simulink model "bus"  (R2020a)
settings: Solver=ode45  StartTime=0.0  StopTime=10.0  RelTol=1e-3
settings Model: Creator=11973  LastModifiedBy=11973

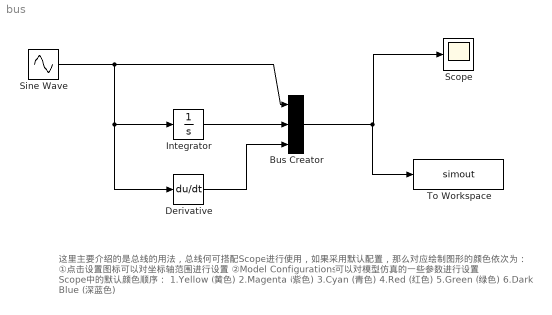
== system bus ==
  note: 这里主要介绍的是总线的用法，总线何可搭配Scope进行使用，如果采用默认配置，那么对应绘制图形的颜色依次为：
      | ①点击设置图标可以对坐标轴范围进行设置
      | ②Model Configurations可以对模型仿真的一些参数进行设置
      | Scope中的默认颜色顺序：
      | 1.Yellow (黄色) 2.Magenta (紫色) 3.Cyan (青色) 4.Red (红色) 5.Green (绿色) 6.Dark Blue (深蓝色)
  Bus Creator : BusCreator  Inputs=3
  Derivative : Derivative
  Integrator : Integrator
  Scope : Scope
  Sine Wave : Sin  SampleTime=0
  To Workspace : ToWorkspace  VariableName=simout  SaveFormat=Timeseries  SampleTime=-1
  wires:
  Sine Wave/1 -> Derivative/1, Integrator/1, Bus Creator/1
  Integrator/1 -> Bus Creator/2
  Derivative/1 -> Bus Creator/3
  Bus Creator/1 -> To Workspace/1, Scope/1
